simulink model "sf_elevator"  (Simulink 6.0)
settings: Solver=ode45  StartTime=0.0  StopTime=inf  RelTol=1e-3
StopFcn:
  | sf_elevator_gui('close');
CloseFcn:
  | sf_elevator_gui('close');
settings Model: CovMetricSettings=dcmtr  Creator=The MathWorks Inc.  LastModifiedBy=batserve  ExtModeAutoUpdateStatusClock=off
settings DataIOCC: SignalLoggingName=sigsOut
settings DebuggingCC: CheckExecutionContextPreStartOutputMsg=on  CheckExecutionContextRuntimeOutputMsg=on  SolverPrmCheckMsg=none
settings HardwareCC: TargetUnknown=on

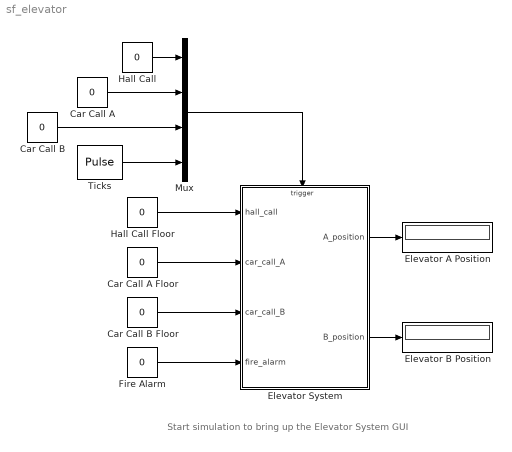
== system sf_elevator ==
  note: Start simulation to bring up the Elevator System GUI
  Car Call A : Constant  Value=0
  Car Call A Floor : Constant  Value=0
  Car Call B : Constant  Value=0
  Car Call B Floor : Constant  Value=0
  Elevator A Position : Display
  Elevator B Position : Display
  Elevator System : Stateflow chart  PropExecContextAcrossSSBoundary=on
  Fire Alarm : Constant  Value=0
  Hall Call : Constant  Value=0
  Hall Call Floor : Constant  Value=0
  Mux : Mux
  Ticks : DiscretePulseGenerator  PulseType=Time based  PulseWidth=50
  wires:
  Hall Call Floor/1 -> Elevator System/1(hall_call)
  Hall Call/1 -> Mux/1
  Mux/1 -> Elevator System/Trigger
  Elevator System/1(A_position) -> Elevator A Position/1
  Elevator System/2(B_position) -> Elevator B Position/1
  Car Call A Floor/1 -> Elevator System/2(car_call_A)
  Car Call B Floor/1 -> Elevator System/3(car_call_B)
  Ticks/1 -> Mux/4
  Car Call A/1 -> Mux/2
  Car Call B/1 -> Mux/3
  Fire Alarm/1 -> Elevator System/4(fire_alarm)

== stateflow chart Elevator System ==
  state Elevator_Manager [parallel]
    en: ml.sf_elevator_gui("init");
    du: process_hall_call();
    A_position = Elevator_A.get_position();
    B_position = Elevator_B.get_position();
    state process_hall_call() [function]
      (default) -> (junction 74)
      (junction 74) -> (junction 73) : {
          | $ $
          | /* Action 'INIT': Initialization */
          | request_floor = hall_call_queue[0];
          | }
      (junction 73) -> (junction 69) : {
          | $ $
          | /* Condition 'fire_alarm_on': Fire alarm is on */
          | fire_alarm_on = (fire_alarm);
          | }
      (junction 69) -> (junction 54) : {
          | $ $
          | /* Condition 'request_outstanding': There is outstanding request */
          | request_outstanding = (request_floor > 0);
          | }
      (junction 54) -> (junction 53) : {
          | $ $
          | /* Condition 'elevator_A_idle': Elevator A is idle */
          | elevator_A_idle = (Elevator_A.get_status() == IDLE);
          | }
      (junction 53) -> (junction 52) : {
          | $ $
          | /* Condition 'elevator_B_idle': Elevator B is idle */
          | elevator_B_idle = (Elevator_B.get_status() == IDLE);
          | }
      (junction 52) -> (junction 51) : {
          | $ $
          | /* Condition 'elevator_A_closer': Elevator A is closer to request */
          | elevator_A_closer = (fabs(Elevator_A.get_position() - request_floor) <= fabs(Elevator_B.get_position() - request_floor));
          | }
      (junction 51) -> (junction 75) : [fire_alarm_on]   /* D1 */
      (junction 75) -> (junction 76) : {
          | $ $
          | /* Action 'EMR': Emergency */
          | Elevator_A.register(floor(Elevator_A.get_position()+Elevator_A.get_direction()/2));
          | Elevator_B.register(floor(Elevator_B.get_position()+Elevator_B.get_direction()/2));
          | }
      (junction 83) -> (junction 80)
      (junction 82) -> (junction 81) : {
          | $ $
          | /* Action 'B': Elevator B should respond to request */
          | Elevator_B.enqueue(request_floor);
          | dequeue(request_floor);
          | }
      (junction 83) -> (junction 82) : [elevator_A_idle&&elevator_B_idle&&!elevator_A_closer]   /* D7 */
      (junction 86) -> (junction 83)
      (junction 85) -> (junction 84) : {
          | $ $
          | /* Action 'A': Elevator A should respond to request */
          | Elevator_A.enqueue(request_floor);
          | dequeue(request_floor);
          | }
      (junction 86) -> (junction 85) : [elevator_A_idle&&elevator_B_idle&&elevator_A_closer]   /* D6 */
      (junction 89) -> (junction 86)
      (junction 88) -> (junction 87) : {
          | $ $
          | /* Action 'B': Elevator B should respond to request */
          | Elevator_B.enqueue(request_floor);
          | dequeue(request_floor);
          | }
      (junction 89) -> (junction 88) : [!elevator_A_idle&&elevator_B_idle]   /* D5 */
      (junction 92) -> (junction 89)
      (junction 91) -> (junction 90) : {
          | $ $
          | /* Action 'A': Elevator A should respond to request */
          | Elevator_A.enqueue(request_floor);
          | dequeue(request_floor);
          | }
      (junction 92) -> (junction 91) : [elevator_A_idle&&!elevator_B_idle]   /* D4 */
      (junction 51) -> (junction 120)
      (junction 120) -> (junction 97) : [!request_outstanding]   /* D2 */
      (junction 97) -> (junction 96) : {
          | $ $
          | /* Action 'NONE': Both elevators are busy, OR no request present */
          |
          | }
      (junction 120) -> (junction 95)
      (junction 95) -> (junction 94) : [!elevator_A_idle&&!elevator_B_idle]   /* D3 */
      (junction 94) -> (junction 93) : {
          | $ $
          | /* Action 'NONE': Both elevators are busy, OR no request present */
          |
          | }
      (junction 95) -> (junction 92)
    state deregister(hall_call_floor) [function]
      (default) -> (junction 104) : {dequeue(hall_call_floor);
          | hall_call_status[hall_call_floor] = 0;
          | ml.sf_elevator_gui("deactivate","hall", hall_call_floor);}
    state enqueue(hall_call_floor) [function]
      (junction 49) -> (junction 48) : [hall_call_status[hall_call_floor] != 0]
      (default) -> (junction 49)
      (junction 64) -> (junction 59) : [i >= NUM_FLOOR]
      (junction 64) -> (junction 60) : {hall_call_queue[i] = hall_call_floor;}
      (junction 66) -> (junction 64)
      (junction 66) -> (junction 66) : [hall_call_queue[i] > 0 && i<NUM_FLOOR]{i++;}
      (junction 66) -> (junction 65) : [hall_call_queue[i] == hall_call_floor]
      (junction 49) -> (junction 66) : {i = 0;}
    state dequeue(hall_call_floor) [function]
      (junction 44) -> (junction 38)
      (junction 44) -> (junction 43) : [i >= NUM_FLOOR || hall_call_queue[i] == 0]
      (junction 63) -> (junction 63) : [hall_call_queue[i] > 0 && ...
          | i<NUM_FLOOR && ...
          | hall_call_queue[i] != hall_call_floor]{i++;}
      (junction 63) -> (junction 44)
      (default) -> (junction 63) : {i=0;}
      (junction 38) -> (junction 62) : {hall_call_queue[i] = hall_call_queue[i+1]; i++;}
      (junction 62) -> (junction 38) : [i < NUM_FLOOR]
      (junction 62) -> (junction 106)
    state register(hall_call_floor) [function]
      (default) -> (junction 101) : {enqueue(hall_call_floor);
          | hall_call_status[hall_call_floor] = 1;}
    state ans = exists_in_queue(floor) [function]
      (junction 135) -> (junction 133) : {ans = i+1;}
      (junction 136) -> (junction 136) : [hall_call_queue[i] > 0 && ...
          | i<NUM_FLOOR && ...
          | hall_call_queue[i] != floor]{i++;}
      (junction 136) -> (junction 135)
      (junction 135) -> (junction 134) : [i >= NUM_FLOOR || hall_call_queue[i] == 0]{ans = 0;}
      (default) -> (junction 136) : {i=0;}
    Elevator_Manager -> (junction 70) : CAR_CALL_B{Elevator_B.register(car_call_B);}
    Elevator_Manager -> (junction 71) : CAR_CALL_A{Elevator_A.register(car_call_A);}
    Elevator_Manager -> (junction 61) : HALL_CALL{register(hall_call);}
  state Elevator_A [parallel]
    state stat = get_status() [function]
      (default) -> (junction 41) : {stat = status;}
    state pos = get_position() [function]
      (default) -> (junction 42) : {pos = position;}
    state register(car_call_floor) [function]
      (default) -> (junction 102) : {enqueue(car_call_floor);
          | car_call_status[car_call_floor] = 1;}
    state deregister(car_call_floor) [function]
      (default) -> (junction 103) : {dequeue(car_call_floor);
          | car_call_status[car_call_floor] = 0;
          | ml.sf_elevator_gui("deactivate","carA",car_call_floor);}
    state Idle
      en: status = IDLE;
      ex: status = BUSY;
    state dequeue(task_floor) [function]
      (junction 39) -> (junction 67) : [i >= NUM_FLOOR || task_queue[i] == 0]
      (junction 40) -> (junction 39)
      (junction 40) -> (junction 40) : [task_queue[i] > 0 && ...
          | i<NUM_FLOOR && ...
          | task_queue[i] != task_floor]{i++;}
      (default) -> (junction 40) : {i=0;}
      (junction 39) -> (junction 68)
      (junction 68) -> (junction 50) : {task_queue[i] = task_queue[i+1]; i++;}
      (junction 50) -> (junction 68) : [i < NUM_FLOOR]
      (junction 50) -> (junction 105)
    state MoveToTask
      du: move_to(task_queue[0]);
    state PickUpDropOff
      en: Elevator_Manager.deregister(cur_floor);
      deregister(cur_floor);
      direction = MOVE_IDLE;
      ml.sf_elevator_gui("open_door","carA");
      du: Elevator_Manager.deregister(cur_floor);
      deregister(cur_floor);
      ex: ml.sf_elevator_gui("close_door","carA");
      state Stopped
      Elevator_A.PickUpDropOff.Stopped -> Elevator_A.PickUpDropOff.Stopped : [fire_alarm]{status = EMERG;}
          | /* Resets the timeout counter */
    state move_to(destination) [function]
      (junction 141) -> (junction 138)
      (junction 140) -> (junction 139) : {
          | $ $
          | /* Action 2: Move down */
          | position = position - VELOCITY;
          | direction = MOVE_DOWN;
          | ml.sf_elevator_gui("move_car", "carA", position);
          | }
      (junction 141) -> (junction 140) : [!move_up&&move_down]   /* D2 */
      (junction 144) -> (junction 141)
      (junction 143) -> (junction 142) : {
          | $ $
          | /* Action 1: Move up */
          | position = position + VELOCITY;
          | direction = MOVE_UP;
          | ml.sf_elevator_gui("move_car", "carA", position);
          | }
      (junction 144) -> (junction 143) : [move_up&&!move_down]   /* D1 */
      (junction 145) -> (junction 144) : {
          | $ $
          | /* Condition 'move_down': Move down */
          | move_down = (position - destination > ERR_TOR);
          | }
      (junction 146) -> (junction 145) : {
          | $ $
          | /* Condition 'move_up': Move up */
          | move_up = (destination - position > ERR_TOR);
          | }
      (default) -> (junction 146)
    state enqueue(task_floor) [function]
      (junction 47) -> (junction 46) : [car_call_status[task_floor] != 0]
      (default) -> (junction 47)
      (junction 56) -> (junction 45) : {task_queue[i] = task_floor;}
      (junction 56) -> (junction 55) : [i >= NUM_FLOOR]
      (junction 57) -> (junction 56)
      (junction 57) -> (junction 57) : [task_queue[i] > 0 && i<NUM_FLOOR]{i++;}
      (junction 57) -> (junction 58) : [task_queue[i] == task_floor]
      (junction 47) -> (junction 57) : {i = 0;}
    state ans = should_stop() [function]
      (junction 127) -> (junction 126) : {
          | $ $
          | /* Condition 'this_hall_call_outstanding': This hall call is still outstanding in queue */
          | this_hall_call_outstanding = (Elevator_Manager.exists_in_queue(cur_floor));
          | }
      (junction 126) -> (junction 125) : [at_destination]   /* D1 */
      (junction 125) -> (junction 124) : {
          | $ $
          | /* Action 'S': Should stop at this floor */
          | position = cur_floor; /* Adjust position */
          | ans = 1;
          | }
      (junction 126) -> (junction 123)
      (junction 123) -> (junction 122) : [!at_a_floor]   /* D2 */
      (junction 122) -> (junction 121) : {
          | $ $
          | /* Action 'C': Should not stop, continue */
          | ans = 0;
          | }
      (junction 123) -> (junction 77)
      (junction 77) -> (junction 78) : [request_from_car]   /* D3 */
      (junction 99) -> (junction 98) : {
          | $ $
          | /* Action 'C': Should not stop, continue */
          | ans = 0;
          | }
      (junction 100) -> (junction 99) : /* Default */
      (junction 109) -> (junction 100)
      (junction 108) -> (junction 107) : {
          | $ $
          | /* Action 'S': Should stop at this floor */
          | position = cur_floor; /* Adjust position */
          | ans = 1;
          | }
      (junction 109) -> (junction 108) : [request_from_hall&&this_hall_call_outstanding]   /* D4 */
      (junction 77) -> (junction 109)
      (junction 78) -> (junction 110) : {
          | $ $
          | /* Action 'S': Should stop at this floor */
          | position = cur_floor; /* Adjust position */
          | ans = 1;
          | }
      (junction 128) -> (junction 127) : {
          | $ $
          | /* Condition 'request_from_hall': There is hall call from this floor */
          | request_from_hall = (Elevator_Manager.hall_call_status[cur_floor]);
          | }
      (junction 129) -> (junction 128) : {
          | $ $
          | /* Condition 'request_from_car': There is car call to stop at this floor */
          | request_from_car = (car_call_status[cur_floor]);
          | }
      (junction 130) -> (junction 129) : {
          | $ $
          | /* Condition 'at_a_floor': Arrived a floor */
          | at_a_floor = (fabs(position - cur_floor) < ERR_TOR);
          | }
      (junction 131) -> (junction 130) : {
          | $ $
          | /* Condition 'at_destination': Arrived destination */
          | at_destination = (fabs(position - task_queue[0]) < ERR_TOR);
          | }
      (junction 132) -> (junction 131) : {
          | $ $
          | /* Action 'INIT': Initialization */
          | cur_floor = ml.round(position);
          | }
      (default) -> (junction 132)
    state dir = get_direction() [function]
      (default) -> (junction 79) : {dir = direction;}
    Elevator_A.Idle -> Elevator_A.MoveToTask : [task_queue[0]]
    Elevator_A.MoveToTask -> Elevator_A.PickUpDropOff : [should_stop()]
    Elevator_A.PickUpDropOff.Stopped -> (junction 72) : after(TIME_OUT, CLOCK)
    (default) -> Elevator_A.Idle
    (junction 72) -> Elevator_A.MoveToTask : [task_queue[0]]
    (junction 72) -> Elevator_A.Idle
  state Elevator_B [parallel]
    state PickUpDropOff
      en: Elevator_Manager.deregister(cur_floor);
      deregister(cur_floor);
      direction = MOVE_IDLE;
      ml.sf_elevator_gui("open_door","carB");
      du: Elevator_Manager.deregister(cur_floor);
      deregister(cur_floor);
      ex: ml.sf_elevator_gui("close_door","carB");
      state Stopped
      Elevator_B.PickUpDropOff.Stopped -> Elevator_B.PickUpDropOff.Stopped : [fire_alarm]{status = EMERG;}
          | /* Resets the timeout counter */
    state Idle
      en: status = IDLE;
      ex: status = BUSY;
    state MoveToTask
      du: move_to(task_queue[0]);
    state move_to(destination) [function]
      (default) -> (junction 177)
      (junction 177) -> (junction 178) : {
          | $ $
          | /* Condition 'move_up': Move up */
          | move_up = (destination - position > ERR_TOR);
          | }
      (junction 178) -> (junction 179) : {
          | $ $
          | /* Condition 'move_down': Move down */
          | move_down = (position - destination > ERR_TOR);
          | }
      (junction 179) -> (junction 180) : [move_up&&!move_down]   /* D1 */
      (junction 180) -> (junction 181) : {
          | $ $
          | /* Action 1: Move up */
          | position = position + VELOCITY;
          | direction = MOVE_UP;
          | ml.sf_elevator_gui("move_car", "carB", position);
          | }
      (junction 179) -> (junction 182)
      (junction 182) -> (junction 183) : [!move_up&&move_down]   /* D2 */
      (junction 183) -> (junction 184) : {
          | $ $
          | /* Action 2: Move down */
          | position = position - VELOCITY;
          | direction = MOVE_DOWN;
          | ml.sf_elevator_gui("move_car", "carB", position);
          | }
      (junction 182) -> (junction 185)
    state ans = should_stop() [function]
      (default) -> (junction 147)
      (junction 147) -> (junction 148) : {
          | $ $
          | /* Action 'INIT': Initialization */
          | cur_floor = ml.round(position);
          | }
      (junction 148) -> (junction 149) : {
          | $ $
          | /* Condition 'at_destination': Arrived destination */
          | at_destination = (fabs(position - task_queue[0]) < ERR_TOR);
          | }
      (junction 149) -> (junction 150) : {
          | $ $
          | /* Condition 'at_a_floor': Arrived a floor */
          | at_a_floor = (fabs(position - cur_floor) < ERR_TOR);
          | }
      (junction 150) -> (junction 151) : {
          | $ $
          | /* Condition 'request_from_car': There is car call to stop at this floor */
          | request_from_car = (car_call_status[cur_floor]);
          | }
      (junction 151) -> (junction 152) : {
          | $ $
          | /* Condition 'request_from_hall': There is hall call from this floor */
          | request_from_hall = (Elevator_Manager.hall_call_status[cur_floor]);
          | }
      (junction 152) -> (junction 153) : {
          | $ $
          | /* Condition 'this_hall_call_outstanding': This hall call is still outstanding in queue */
          | this_hall_call_outstanding = (Elevator_Manager.exists_in_queue(cur_floor));
          | }
      (junction 153) -> (junction 154) : [at_destination]   /* D1 */
      (junction 154) -> (junction 155) : {
          | $ $
          | /* Action 'S': Should stop at this floor */
          | position = cur_floor; /* Adjust position */
          | ans = 1;
          | }
      (junction 153) -> (junction 156)
      (junction 156) -> (junction 157) : [!at_a_floor]   /* D2 */
      (junction 157) -> (junction 158) : {
          | $ $
          | /* Action 'C': Should not stop, continue */
          | ans = 0;
          | }
      (junction 156) -> (junction 159)
      (junction 159) -> (junction 160) : [request_from_car]   /* D3 */
      (junction 160) -> (junction 161) : {
          | $ $
          | /* Action 'S': Should stop at this floor */
          | position = cur_floor; /* Adjust position */
          | ans = 1;
          | }
      (junction 159) -> (junction 162)
      (junction 162) -> (junction 163) : [request_from_hall&&this_hall_call_outstanding]   /* D4 */
      (junction 163) -> (junction 164) : {
          | $ $
          | /* Action 'S': Should stop at this floor */
          | position = cur_floor; /* Adjust position */
          | ans = 1;
          | }
      (junction 162) -> (junction 165)
      (junction 165) -> (junction 166) : /* Default */
      (junction 166) -> (junction 167) : {
          | $ $
          | /* Action 'C': Should not stop, continue */
          | ans = 0;
          | }
    state dir = get_direction() [function]
      (default) -> (junction 168) : {dir = direction;}
    state register(car_call_floor) [function]
      (default) -> (junction 169) : {enqueue(car_call_floor);
          | car_call_status[car_call_floor] = 1;}
    state enqueue(task_floor) [function]
      (default) -> (junction 170)
      (junction 170) -> (junction 171) : [car_call_status[task_floor] != 0]
      (junction 170) -> (junction 173) : {i = 0;}
      (junction 173) -> (junction 172) : [task_queue[i] == task_floor]
      (junction 173) -> (junction 173) : [task_queue[i] > 0 && i<NUM_FLOOR]{i++;}
      (junction 173) -> (junction 174)
      (junction 174) -> (junction 175) : [i >= NUM_FLOOR]
      (junction 174) -> (junction 176) : {task_queue[i] = task_floor;}
    state pos = get_position() [function]
      (default) -> (junction 119) : {pos = position;}
    state deregister(car_call_floor) [function]
      (default) -> (junction 118) : {dequeue(car_call_floor);
          | car_call_status[car_call_floor] = 0;
          | ml.sf_elevator_gui("deactivate","carB",car_call_floor);}
    state stat = get_status() [function]
      (default) -> (junction 117) : {stat = status;}
    state dequeue(task_floor) [function]
      (junction 112) -> (junction 111)
      (junction 112) -> (junction 113) : [i < NUM_FLOOR]
      (junction 113) -> (junction 112) : {task_queue[i] = task_queue[i+1]; i++;}
      (junction 115) -> (junction 113)
      (junction 115) -> (junction 114) : [i >= NUM_FLOOR || task_queue[i] == 0]
      (junction 116) -> (junction 115)
      (junction 116) -> (junction 116) : [task_queue[i] > 0 && ...
          | i<NUM_FLOOR && ...
          | task_queue[i] != task_floor]{i++;}
      (default) -> (junction 116) : {i=0;}
    (default) -> Elevator_B.Idle
    (junction 137) -> Elevator_B.Idle
    Elevator_B.PickUpDropOff.Stopped -> (junction 137) : after(TIME_OUT, CLOCK)
    (junction 137) -> Elevator_B.MoveToTask : [task_queue[0]]
    Elevator_B.Idle -> Elevator_B.MoveToTask : [task_queue[0]]
    Elevator_B.MoveToTask -> Elevator_B.PickUpDropOff : [should_stop()]
  data: request_floor temporary uint8; fire_alarm_on temporary boolean; request_outstanding temporary boolean; elevator_A_idle temporary boolean; elevator_B_idle temporary boolean; elevator_A_closer temporary boolean; hall_call_queue local uint8 size=10; hall_call_status local uint8 size=10; status local uint8; position local double =1; task_queue local uint8 size=10; car_call_status local uint8 size=10; car_call local uint8; cur_floor local uint8; direction local uint8 =1; stat function_output uint8; pos function_output double; car_call_floor function_input uint8; hall_call_floor function_input uint8; car_call_floor function_input uint8; i temporary uint8; task_floor function_input uint8; hall_call_floor function_input uint8; i temporary uint8; destination function_input double; move_up temporary boolean; move_down temporary boolean; i temporary uint8; hall_call_floor function_input uint8; task_floor function_input uint8; i temporary uint8; hall_call_floor function_input uint8; ans function_output boolean; at_destination temporary boolean; at_a_floor temporary boolean; request_from_car temporary boolean; request_from_hall temporary boolean; this_hall_call_outstanding temporary boolean; dir function_output uint8; ans function_output uint8; floor function_input uint8; i temporary uint8; status local uint8; position local double =1; task_queue local uint8 size=10; car_call_status local uint8 size=10; car_call local uint8; cur_floor local uint8; direction local uint8 =1; destination function_input double; move_up temporary boolean; move_down temporary boolean; ans function_output boolean; at_destination temporary boolean; at_a_floor temporary boolean; request_from_car temporary boolean; request_from_hall temporary boolean; this_hall_call_outstanding temporary boolean; dir function_output uint8; car_call_floor function_input uint8; task_floor function_input uint8; i temporary uint8; pos function_output double; car_call_floor function_input uint8; stat function_output uint8; i temporary uint8; task_floor function_input uint8; IDLE constant uint8; BUSY constant uint8 =1; VELOCITY local double =0.01; hall_call input uint8; A_position output double =1; B_position output double =1; NUM_FLOOR constant uint8 =9; ERR_TOR local double =0.001; car_call_A input uint8; car_call_B input uint8; fire_alarm input uint8; MOVE_UP constant uint8 =2; MOVE_DOWN constant uint8; MOVE_IDLE constant uint8 =1; EMERG constant uint8 =2; TIME_OUT constant uint32 =1000
  data fire_alarm_on settings: description=Fire alarm is on
  data request_outstanding settings: description=There is outstanding request
  data elevator_A_idle settings: description=Elevator A is idle
  data elevator_B_idle settings: description=Elevator B is idle
  data elevator_A_closer settings: description=Elevator A is closer to request
  data move_up settings: description=Move up
  data move_down settings: description=Move down
  data at_destination settings: description=Arrived destination
  data at_a_floor settings: description=Arrived a floor
  data request_from_car settings: description=There is car call to stop at this floor
  data request_from_hall settings: description=There is hall call from this floor
  data this_hall_call_outstanding settings: description=This hall call is still outstanding in queue
  data move_up settings: description=Move up
  data move_down settings: description=Move down
  data at_destination settings: description=Arrived destination
  data at_a_floor settings: description=Arrived a floor
  data request_from_car settings: description=There is car call to stop at this floor
  data request_from_hall settings: description=There is hall call from this floor
  data this_hall_call_outstanding settings: description=This hall call is still outstanding in queue
  events: HALL_CALL input EITHER_EDGE_EVENT; CAR_CALL_A input EITHER_EDGE_EVENT; CAR_CALL_B input EITHER_EDGE_EVENT; CLOCK input EITHER_EDGE_EVENT
